simulink model "disco_f407_Interrupt_push_button"  (R2015a)
settings: Solver=FixedStepDiscrete  SolverMode=SingleTasking  StartTime=0.0  StopTime=10.0  FixedStep=1e-3  RelTol=1e-3
libraries: mbed_lib x3
settings Model: CovSFcnEnable=off  Creator=oh  LastModifiedBy=oh
settings OptimizationCC: OptimizeModelRefInitCode=on  LifeSpan=1
settings DebuggingCC: SolverPrmCheckMsg=warning
settings HardwareCC: ProdLargestAtomicInteger=Long  ProdLargestAtomicFloat=Double  ProdEndianess=LittleEndian  ProdHWDeviceType=ARM Compatible->ARM Cortex
settings RTWCC: SystemTargetFile=mbed.tlc  TemplateMakefile=mbed.tmf  Description=Mbed Target (Embedded Target)  TargetLang=C++
settings CodeAppCC: IgnoreCustomStorageClasses=off
settings STFCustomTargetCC: CombineOutputUpdateFcns=on  SupportContinuousTime=off  SupportVariableSizeSignals=off  SystemTargetFile=mbed.tlc
settings ERTTargetCC: SupportContinuousTime=off  SupportVariableSizeSignals=off  ERTCustomFileTemplate=mbed_file_process.tlc

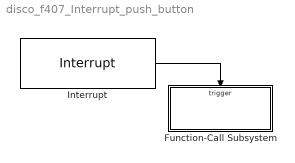
== system disco_f407_Interrupt_push_button ==
  Function-Call Subsystem : Subsystem  TreatAsAtomicUnit=on
  Interrupt : mbed_lib/GPIO/Interrupt  PortName=A  PinNumber=0  Interrupt=Both
  wires:
  Interrupt/1 -> Function-Call Subsystem/Trigger

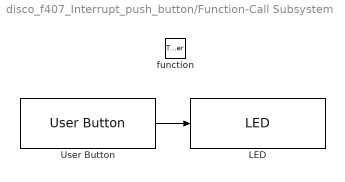
== system disco_f407_Interrupt_push_button/Function-Call Subsystem ==
  function : TriggerPort  TriggerType=function-call
  LED : mbed_lib/GPIO/LED  nLED=1  SampleTime=-1
  User Button : mbed_lib/GPIO/User Button  SampleTime=-1
  wires:
  User Button/1 -> LED/1
